simulink model "PipeIsolation_1"  (Simulink 8.2)
settings: Solver=ode45  StartTime=0.0  StopTime=3600  RelTol=1e-5
undefined symbols (not defined in the file): density
libraries: carnot x5
settings Model: Creator=drhf  LastModifiedBy=drhf

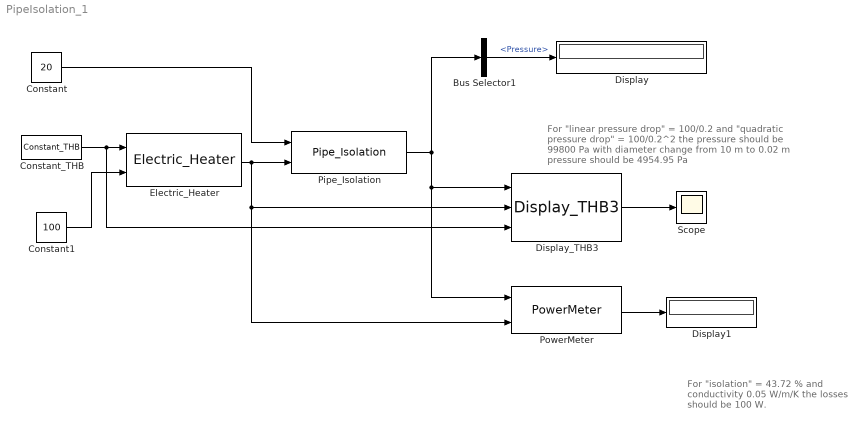
== system PipeIsolation_1 ==
  note: For "isolation" = 43.72 % and
      | conductivity 0.05 W/m/K
      | the losses should be 100 W.
  note: For "linear pressure drop" = 100/0.2
      | and "quadratic pressure drop" = 100/0.2^2
      | the pressure should be 99800 Pa
      | with diameter change from 10 m to 0.02 m
      | pressure should be 4954.95 Pa
  Bus Selector1 : BusSelector  OutputSignals=Pressure
  Constant : Constant  Value=20
  Constant1 : Constant  Value=100
  Constant_THB : carnot/Source/Simple/Constant_THB  t=40  mdot=720/3600  p=1e5  mID=Full Pressure Drop with Static Height  fluid=Water  mix=0  dia=10  hgt=0
  Display : Display
      settings: Format=decimal (Stored Integer)
  Display1 : Display
  Display_THB3 : carnot/Outputs/Display_THB3  t=on  m=off  p=off  id=off  mix=off  d=off
  Electric_Heater : carnot/Source/Boiler/Electric_Heater
  Pipe_Isolation : carnot/Hydraulics/Pipe_Isolation  dia=0.02  len=10  hgt=5e4/(9.81*density(40.0536031,2e5,1,0))  isolat=43.72  condiso=0.05  cond=0  cwall=1000  t0=20  lin=100/0.2  qua=100/0.2^2  nodes=10
  PowerMeter : carnot/Control/PowerMeter
  Scope : Scope
      settings: TimeRange=4000  YMin=39.66951326595616  YMax=40.42277164649369
  wires:
  Constant/1 -> Pipe_Isolation/1
  Pipe_Isolation/1 -> Bus Selector1/1, Display_THB3/1, PowerMeter/1
  Bus Selector1/1 -> Display/1  "<Pressure>"
  Constant_THB/1 -> Display_THB3/3, Electric_Heater/1
  Electric_Heater/1 -> Display_THB3/2, PowerMeter/2, Pipe_Isolation/2
  Constant1/1 -> Electric_Heater/2
  Display_THB3/1 -> Scope/1
  PowerMeter/1 -> Display1/1
